simulink model "rr_adaptive_computedTorque"  (R2024b)
settings: Solver=FixedStepAuto  StartTime=0.0  StopTime=200  FixedStep=0.001  MaxStep=0.001  RelTol=1e-12  AbsTol=1e-9
undefined symbols (not defined in the file): dq0, dq0_d, p_0, p_real, par_nl, q0, q0_d
settings Model: Creator=Mathew  LastModifiedBy=aldos
settings SolverCC: AlgebraicLoopSolver=TrustRegion
settings DebuggingCC: UnconnectedInputMsg=warning  UnconnectedOutputMsg=warning  UnconnectedLineMsg=warning
settings ModelReferenceCC: EnableRefExpFcnMdlSchedulingChecks=on
settings SFSimCC: CustomCodeUndefinedFunction=UseInterfaceOnly
settings RTWCC: GPUComputeCapability=3.5  DLArmComputeVersion=19.05

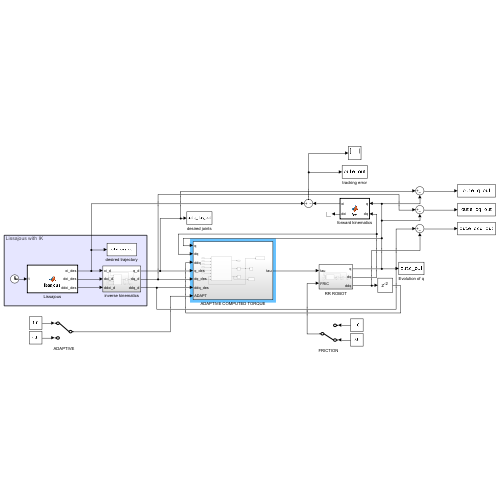
[thumbnail: Simulink's stored preview of the top-level diagram]
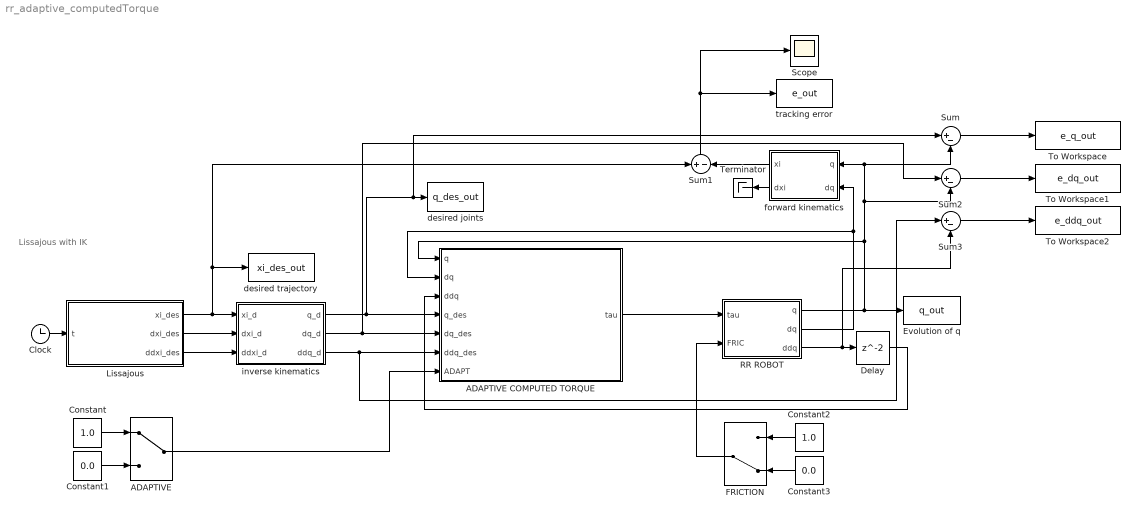
== system rr_adaptive_computedTorque ==
  note: Lissajous with IK
  ADAPTIVE : ManualSwitch
  ADAPTIVE COMPUTED TORQUE : Subsystem
  Clock : Clock
  Constant : Constant  Value=1.0
  Constant1 : Constant  Value=0.0
  Constant2 : Constant  Value=1.0
  Constant3 : Constant  Value=0.0
  Delay : Delay
  Evolution of q : ToWorkspace  VariableName=q_out  SaveFormat=Timeseries  SampleTime=-1
  FRICTION : ManualSwitch  CurrentSetting=0
  Lissajous : MATLAB Function  TreatAsAtomicUnit=on
  RR ROBOT : Subsystem
  Scope : Scope
  Sum : Sum  Inputs=|+-
  Sum1 : Sum  Inputs=+-
  Sum2 : Sum  Inputs=|+-
  Sum3 : Sum  Inputs=|+-
  Terminator : Terminator
  To Workspace : ToWorkspace  VariableName=e_q_out  SaveFormat=Timeseries  SampleTime=-1
  To Workspace1 : ToWorkspace  VariableName=e_dq_out  SaveFormat=Timeseries  SampleTime=-1
  To Workspace2 : ToWorkspace  VariableName=e_ddq_out  SaveFormat=Timeseries  SampleTime=-1
  desired joints : ToWorkspace  VariableName=q_des_out  SaveFormat=Timeseries  SampleTime=-1
  desired trajectory : ToWorkspace  VariableName=xi_des_out  SaveFormat=Timeseries  SampleTime=-1
  forward kinematics : MATLAB Function  TreatAsAtomicUnit=on
  inverse kinematics : Subsystem
  tracking error : ToWorkspace  VariableName=e_out  SaveFormat=Timeseries  SampleTime=-1
  wires:
  RR ROBOT/1(q) -> Sum2/2, Sum/2, forward kinematics/1(q), ADAPTIVE COMPUTED TORQUE/1(q), Evolution of q/1
  RR ROBOT/2(dq) -> forward kinematics/2(dq), ADAPTIVE COMPUTED TORQUE/2(dq)
  inverse kinematics/1(q_d) -> ADAPTIVE COMPUTED TORQUE/4(q_des), Sum/1, desired joints/1
  Clock/1 -> Lissajous/1(t)
  Lissajous/2(dxi_des) -> inverse kinematics/2(dxi_d)
  Lissajous/3(ddxi_des) -> inverse kinematics/3(ddxi_d)
  Lissajous/1(xi_des) -> Sum1/1, desired trajectory/1, inverse kinematics/1(xi_d)
  Sum1/1 -> tracking error/1, Scope/1
  ADAPTIVE COMPUTED TORQUE/1(tau) -> RR ROBOT/1(tau)
  forward kinematics/2(dxi) -> Terminator/1
  forward kinematics/1(xi) -> Sum1/2
  inverse kinematics/2(dq_d) -> Sum2/1, ADAPTIVE COMPUTED TORQUE/5(dq_des)
  inverse kinematics/3(ddq_d) -> Sum3/1, ADAPTIVE COMPUTED TORQUE/6(ddq_des)
  Constant/1 -> ADAPTIVE/1
  Constant1/1 -> ADAPTIVE/2
  ADAPTIVE/1 -> ADAPTIVE COMPUTED TORQUE/7(ADAPT)
  FRICTION/1 -> RR ROBOT/2(FRIC)
  Constant2/1 -> FRICTION/1
  Constant3/1 -> FRICTION/2
  RR ROBOT/3(ddq) -> Sum3/2, Delay/1
  Delay/1 -> ADAPTIVE COMPUTED TORQUE/3(ddq)
  Sum3/1 -> To Workspace2/1
  Sum2/1 -> To Workspace1/1
  Sum/1 -> To Workspace/1

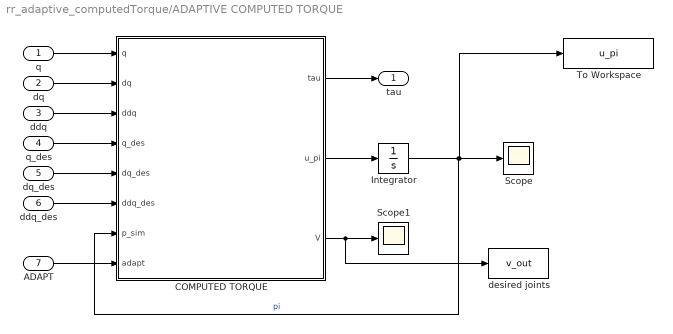
== system rr_adaptive_computedTorque/ADAPTIVE COMPUTED TORQUE ==
  q : Inport
  dq : Inport  Port=2
  ddq : Inport  Port=3
  q_des : Inport  Port=4
  dq_des : Inport  Port=5
  ddq_des : Inport  Port=6
  ADAPT : Inport  Port=7
  COMPUTED TORQUE : MATLAB Function  TreatAsAtomicUnit=on
  Integrator : Integrator  InitialCondition=p_0
  Scope : Scope
  Scope1 : Scope
  To Workspace : ToWorkspace  VariableName=u_pi  SaveFormat=Timeseries  SampleTime=-1
  desired joints : ToWorkspace  VariableName=v_out  SaveFormat=Timeseries  SampleTime=-1
  tau : Outport
  wires:
  ddq_des/1 -> COMPUTED TORQUE/6(ddq_des)
  dq/1 -> COMPUTED TORQUE/2(dq)
  COMPUTED TORQUE/1(tau) -> tau/1
  q_des/1 -> COMPUTED TORQUE/4(q_des)
  q/1 -> COMPUTED TORQUE/1(q)
  dq_des/1 -> COMPUTED TORQUE/5(dq_des)
  COMPUTED TORQUE/2(u_pi) -> Integrator/1
  Integrator/1 -> COMPUTED TORQUE/7(p_sim), To Workspace/1, Scope/1  "pi"
  ddq/1 -> COMPUTED TORQUE/3(ddq)
  ADAPT/1 -> COMPUTED TORQUE/8(adapt)
  COMPUTED TORQUE/3(V) -> desired joints/1, Scope1/1

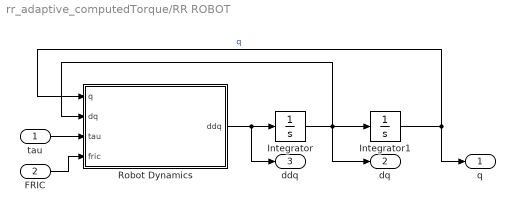
== system rr_adaptive_computedTorque/RR ROBOT ==
  tau : Inport
  FRIC : Inport  Port=2
  Integrator : Integrator  InitialCondition=dq0
  Integrator1 : Integrator  InitialCondition=q0
  Robot Dynamics : MATLAB Function  TreatAsAtomicUnit=on
  q : Outport  PortDimensions=[3, 1]
  dq : Outport  Port=2  PortDimensions=[3, 1]
  ddq : Outport  Port=3  PortDimensions=[3, 1]
  wires:
  Robot Dynamics/1(ddq) -> ddq/1, Integrator/1
  Integrator/1 -> Robot Dynamics/2(dq), dq/1, Integrator1/1
  tau/1 -> Robot Dynamics/3(tau)
  Integrator1/1 -> Robot Dynamics/1(q), q/1  "q"
  FRIC/1 -> Robot Dynamics/4(fric)

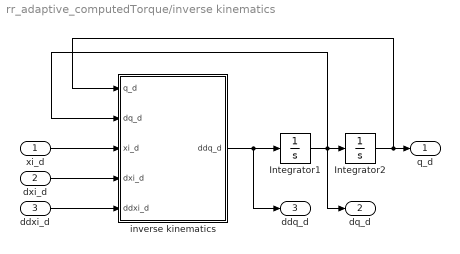
== system rr_adaptive_computedTorque/inverse kinematics ==
  xi_d : Inport
  dxi_d : Inport  Port=2
  ddxi_d : Inport  Port=3
  Integrator1 : Integrator  InitialCondition=dq0_d
  Integrator2 : Integrator  InitialCondition=q0_d
  inverse kinematics : MATLAB Function  TreatAsAtomicUnit=on
  q_d : Outport
  dq_d : Outport  Port=2
  ddq_d : Outport  Port=3
  wires:
  inverse kinematics/1(ddq_d) -> Integrator1/1, ddq_d/1
  Integrator2/1 -> inverse kinematics/1(q_d), q_d/1
  ddxi_d/1 -> inverse kinematics/5(ddxi_d)
  dxi_d/1 -> inverse kinematics/4(dxi_d)
  xi_d/1 -> inverse kinematics/3(xi_d)
  Integrator1/1 -> inverse kinematics/2(dq_d), dq_d/1, Integrator2/1

== matlab function rr_adaptive_computedTorque/ADAPTIVE COMPUTED TORQUE/COMPUTED TORQUE ==
  data: q input; dq input; ddq input; q_des input; dq_des input; ddq_des input; tau output; par_nl parameter; p_sim input; adapt input; u_pi output; V output; p_real parameter
function [tau, u_pi, V] = computed_torque(q, dq, ddq, q_des, dq_des, ddq_des, par_nl, p_sim, adapt, p_real)

% control parameters
kp = 16;
kv = 8;

% Get dynamic matrices
M = get_Mp(q, p_sim, par_nl);
C = get_Cp(q, dq, p_sim, par_nl);
G = get_Gp(q, p_sim, par_nl);

% error computation
e = q_des - q;
de = dq_des - dq;

tau = M*(ddq_des + kv*de + kp*e) + C*dq + G; % + D*dq;    %%COMPUTED TORQUE'S LAW

%% adaptive
coder.extrinsic('lyap');

R = 10*diag([1, 1, 1, 1, 1, 1, 1, 1, 1]);

A_lin = [zeros(3,3), eye(3,3); -kp*eye(3,3), -kv*eye(3,3)];
B_lin = [zeros(3,3); eye(3,3)];
P = zeros(6,6);
Q = eye(6,6);
P = lyap(A_lin', Q);

x = [e; de];
w = B_lin' * P * x;

Y = get_Y(q, dq, dq, ddq, par_nl);

u_pi = R^-1 * Y' * (M^-1)' * w;
u_pi = adapt * u_pi;

%% Lyapunov
e_p = p_real - p_sim;
% V = 1/2*(e')*e + 1/2*(de')*de + 1/2*(e_p')*R*e_p;
V = 1/2*[e;de]'*P*[e;de] + 1/2*(e_p')*R*e_p;

== matlab function rr_adaptive_computedTorque/RR ROBOT/Robot Dynamics ==
  data: q input; dq input; tau input; ddq output; par_real parameter; fric input
function ddq = inverse_dynamics(q, dq, tau, par_real, fric)

% Get dynamic matrices
M = get_M(q, par_real);
C = get_C(q, dq, par_real);
G = get_G(q, par_real);
D = get_D(par_real);

% obtain joint accelerations
ddq = inv(M)*(tau - C*dq - G - fric*D*dq);

== matlab function rr_adaptive_computedTorque/Lissajous ==
  data: t input; xi_des output size=[2,1]; dxi_des output size=[2,1]; ddxi_des output size=[2,1]; par_traj parameter
function [xi_des, dxi_des, ddxi_des] = lissajous(t, par_traj)

A = par_traj.A;
B = par_traj.B;
a = par_traj.a;
b = par_traj.b;
d = par_traj.d;
xi0 = par_traj.xi0;

xi_des = [A*sin(a*t+d); B*sin(b*t)] + xi0;

% xi_des = [A*sin(a*t+d) + 0.3*A*sin(3*a*t);
%           B*sin(b*t)   + 0.3*B*sin(2*b*t+pi/3)] + xi0;

dxi_des = [A*a*cos(a*t+d); B*b*cos(b*t)];
ddxi_des = [-A*a^2*sin(a*t+d); -B*b^2*sin(b*t)];
end

== matlab function rr_adaptive_computedTorque/inverse kinematics/inverse kinematics ==
  data: q_d input; dq_d input; xi_d input; dxi_d input; ddxi_d input; ddq_d output size=[3, 1]; par_kin parameter
function ddq_d = fcn(q_d, dq_d, xi_d, dxi_d, ddxi_d, par_kin)

% jacobian
J_full = get_J(q_d, par_kin);
J = J_full(1:2,:);
% jacobian derivative
J_dot_full = get_J_dot(q_d, dq_d, par_kin);
J_dot = J_dot_full(1:2,:);
% pseudoinverse
pinv_J = pinv(J);
% forward kinematics
[xi_curr, dxi_curr] = RR_forward_kinematics(q_d, dq_d, par_kin);

% second order CLIK
Kp = 100;
Kv = 80;
ddq_d = pinv_J * (ddxi_d - J_dot * dq_d + Kv*(dxi_d-dxi_curr) + Kp*(xi_d-xi_curr));
% ddq_d = pinv_J * ([ddxi_d; 0] - J_dot * dq_d + Kv*([dxi_d;0]-[dxi_curr;0]) + Kp*([xi_d;0]-[xi_curr;0]));

== matlab function rr_adaptive_computedTorque/forward kinematics ==
  data: q input; xi output; dq input; par_kin parameter; dxi output
function [xi, dxi] = fcn(q, dq, par_kin)

[xi, dxi] = RR_forward_kinematics(q, dq, par_kin);

end
